simulink model "controller_modified_Ardiono"  (R2023b)
settings: Solver=FixedStepDiscrete  StartTime=0.0  StopTime=100  FixedStep=1/100  RelTol=1e-3  EnableMultiTasking=on
undefined symbols (not defined in the file): MAX_TORQUE, MAX_TORQUE_REVERSE
libraries: arduinolib x17
settings Model: ExtModeTrigDuration=2  Creator=DAUIN-Win10  LastModifiedBy=RSKALA
settings OptimizationCC: EnhancedBackFolding=on  PassReuseOutputArgsAs=Individual arguments  ZeroExternalMemoryAtStartup=off  ZeroInternalMemoryAtStartup=off  MaxStackSize=64  OptimizeBlockOrder=speed  DifferentSizesBufferReuse=on  OptimizationCustomize=off  EfficientTunableParamExpr=on
settings DebuggingCC: ParameterTunabilityLossMsg=error  UnconnectedInputMsg=warning  UnconnectedOutputMsg=warning  UnconnectedLineMsg=warning
settings HardwareCC: ProdBitPerInt=16  ProdBitPerPointer=16  ProdBitPerSizeT=16  ProdBitPerPtrDiffT=16  ProdLargestAtomicFloat=None  ProdWordSize=8  ProdHWDeviceType=Atmel->AVR
settings ModelReferenceCC: EnableRefExpFcnMdlSchedulingChecks=on
settings SFSimCC: MATLABDynamicMemAlloc=off
settings RTWCC: Description=Embedded Coder  SystemTargetFile=ert.tlc  HardwareBoard=Arduino Uno  TemplateMakefile=ert_default_tmf  Toolchain=Arduino AVR  BuildConfiguration=Faster Runs  DLArmComputeVersion=19.05
settings CodeAppCC: ForceParamTrailComments=on  IgnoreCustomStorageClasses=off  OperatorAnnotations=on  SimulinkDataObjDesc=on  SFDataObjDesc=on  InsertBlockDesc=on
settings ERTTargetCC: SupportContinuousTime=on  SupportVariableSizeSignals=on  ExtModeTransport=3  ExtModeStaticAlloc=on  ExtModeAutomaticAllocSize=off  ExtModeStaticAllocSize=250  ExtModeMexFile=ext_xcp  ExtModeIntrfLevel=Level2 - Open

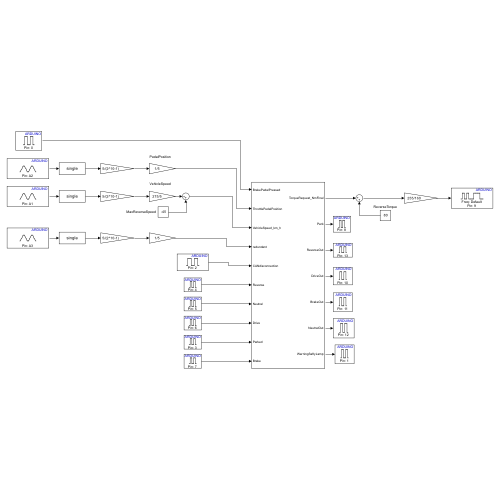
[thumbnail: Simulink's stored preview of the top-level diagram]
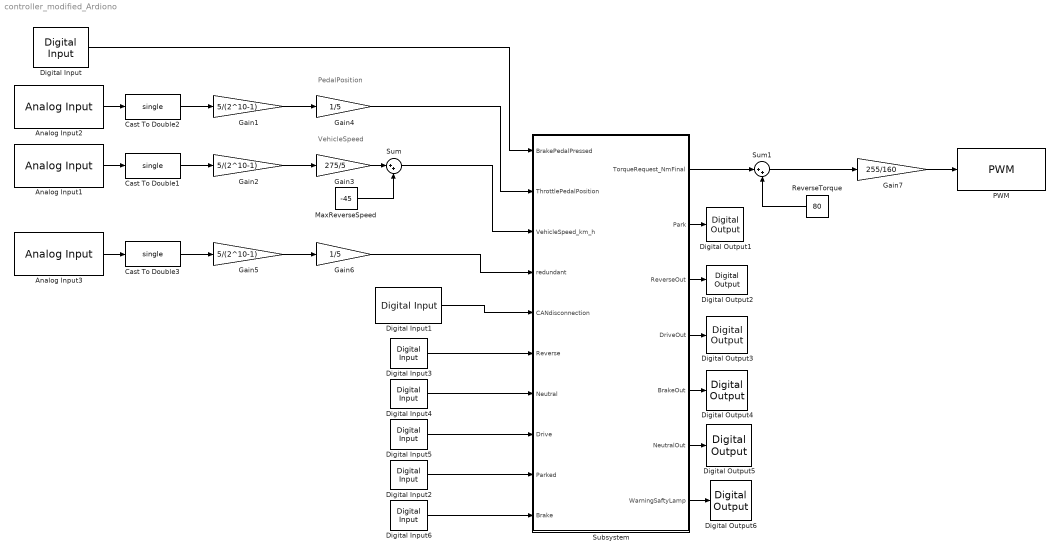
== system controller_modified_Ardiono ==
  note: VehicleSpeed
  note: PedalPosition
  Analog Input1 : arduinolib/Analog Input  pinNumber=1  ReadResultsOnly=off  ConversionTriggerSource=Software  ExternalTriggerType=uint32( 0 )  OutputDataType=uint16  EnableConversionCompleteNotify=off  EnableOuputStatus=off  SampleTime=-1  blockPlatform=arduino
  Analog Input2 : arduinolib/Analog Input  pinNumber=2  ReadResultsOnly=off  ConversionTriggerSource=Software  ExternalTriggerType=uint32( 0 )  OutputDataType=uint16  EnableConversionCompleteNotify=off  EnableOuputStatus=off  SampleTime=-1  blockPlatform=arduino
  Analog Input3 : arduinolib/Analog Input  pinNumber=3  ReadResultsOnly=off  ConversionTriggerSource=Software  ExternalTriggerType=uint32( 0 )  OutputDataType=uint16  EnableConversionCompleteNotify=off  EnableOuputStatus=off  SampleTime=-1  blockPlatform=arduino
  Cast To Double1 : DataTypeConversion  OutDataTypeStr=single  SaturateOnIntegerOverflow=off  RndMeth=Floor
  Cast To Double2 : DataTypeConversion  OutDataTypeStr=single  SaturateOnIntegerOverflow=off  RndMeth=Floor
  Cast To Double3 : DataTypeConversion  OutDataTypeStr=single  SaturateOnIntegerOverflow=off  RndMeth=Floor
  Digital Input : arduinolib/Digital Input  pinNumber=0  mode=Default  Direction=input  SampleTime=0.1  blockPlatform=arduino
  Digital Input1 : arduinolib/Digital Input  pinNumber=2  mode=Default  Direction=input  SampleTime=0.1  blockPlatform=arduino
  Digital Input2 : arduinolib/Digital Input  pinNumber=3  mode=Default  Direction=input  SampleTime=0.1  blockPlatform=arduino
  Digital Input3 : arduinolib/Digital Input  pinNumber=4  mode=Default  Direction=input  SampleTime=0.1  blockPlatform=arduino
  Digital Input4 : arduinolib/Digital Input  pinNumber=5  mode=Default  Direction=input  SampleTime=0.1  blockPlatform=arduino
  Digital Input5 : arduinolib/Digital Input  pinNumber=6  mode=Default  Direction=input  SampleTime=0.1  blockPlatform=arduino
  Digital Input6 : arduinolib/Digital Input  pinNumber=7  mode=Default  Direction=input  SampleTime=0.1  blockPlatform=arduino
  Digital Output1 : arduinolib/Digital Output  pinNumber=8  Direction=output  blockPlatform=arduino
  Digital Output2 : arduinolib/Digital Output  pinNumber=13  Direction=output  blockPlatform=arduino
  Digital Output3 : arduinolib/Digital Output  pinNumber=10  Direction=output  blockPlatform=arduino
  Digital Output4 : arduinolib/Digital Output  pinNumber=11  Direction=output  blockPlatform=arduino
  Digital Output5 : arduinolib/Digital Output  pinNumber=12  Direction=output  blockPlatform=arduino
  Digital Output6 : arduinolib/Digital Output  pinNumber=1  Direction=output  blockPlatform=arduino
  Gain1 : Gain  Gain=5/(2^10-1)
  Gain2 : Gain  Gain=5/(2^10-1)
  Gain3 : Gain  Gain=275/5  OutDataTypeStr=single
  Gain4 : Gain  Gain=1/5
  Gain5 : Gain  Gain=5/(2^10-1)
  Gain6 : Gain  Gain=1/5
  Gain7 : Gain  Gain=255/160
  MaxReverseSpeed : Constant  Value=-45  OutDataTypeStr=single
  PWM : arduinolib/PWM  pinNumber=9  frequencyType=Default  desiredFrequency=490.2  achievableFrequency=490.2
  ReverseTorque : Constant  Value=80
  Subsystem : Subsystem
  Sum : Sum  Inputs=|++  OutDataTypeStr=single
  Sum1 : Sum  Inputs=|++
  wires:
  Cast To Double2/1 -> Gain1/1
  Gain5/1 -> Gain6/1
  Digital Input3/1 -> Subsystem/6(Reverse)
  Analog Input2/1 -> Cast To Double2/1
  Gain2/1 -> Gain3/1
  Gain3/1 -> Sum/1
  MaxReverseSpeed/1 -> Sum/2
  Digital Input4/1 -> Subsystem/7(Neutral)
  Analog Input1/1 -> Cast To Double1/1
  Digital Input5/1 -> Subsystem/8(Drive)
  Analog Input3/1 -> Cast To Double3/1
  Digital Input6/1 -> Subsystem/10(Brake)
  Cast To Double3/1 -> Gain5/1
  Digital Input/1 -> Subsystem/1(BrakePedalPressed)
  Gain4/1 -> Subsystem/2(ThrottlePedalPosition)
  Sum/1 -> Subsystem/3(VehicleSpeed_km_h)
  Cast To Double1/1 -> Gain2/1
  Digital Input2/1 -> Subsystem/9(Parked)
  Gain1/1 -> Gain4/1
  Gain6/1 -> Subsystem/4(redundant)
  Digital Input1/1 -> Subsystem/5(CANdisconnection)
  Sum1/1 -> Gain7/1
  Gain7/1 -> PWM/1
  ReverseTorque/1 -> Sum1/2
  Subsystem/5(BrakeOut) -> Digital Output4/1
  Subsystem/4(DriveOut) -> Digital Output3/1
  Subsystem/3(ReverseOut) -> Digital Output2/1
  Subsystem/2(Park) -> Digital Output1/1
  Subsystem/1(TorqueRequest_NmFinal) -> Sum1/1
  Subsystem/6(NeutralOut) -> Digital Output5/1
  Subsystem/7(WarningSaftyLamp) -> Digital Output6/1

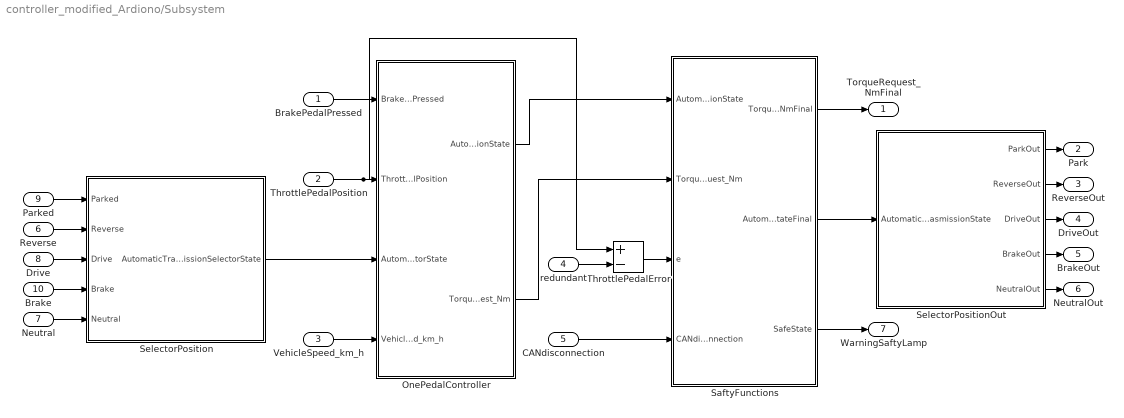
== system controller_modified_Ardiono/Subsystem ==
  BrakePedalPressed : Inport  OutDataTypeStr=boolean
  ThrottlePedalPosition : Inport  Port=2  OutDataTypeStr=single
  VehicleSpeed_km_h : Inport  Port=3  OutDataTypeStr=single  Unit=km/h
  redundant : Inport  Port=4  OutDataTypeStr=single  Unit=km/h
  CANdisconnection : Inport  Port=5
  Reverse : Inport  Port=6
  Neutral : Inport  Port=7
  Drive : Inport  Port=8
  Parked : Inport  Port=9
  Brake : Inport  Port=10
  OnePedalController : Stateflow chart  TreatAsAtomicUnit=on
  SaftyFunctions : Stateflow chart  TreatAsAtomicUnit=on
      settings: PortSchema="{\"entries\":[{\"content\":{\"sides\":[{\"content\":{\"connectorIds\":[\"In1\",\"In2\",\"In4\",\"In3\"]},\"type\":\"ConnectorPlacement.EquallySpacedRectSide\",\"uuid\":\"7fe74ee5-44b1-4d05-a413-f8cbf6cc4146\"},{\"content\":{\"connectorIds\":[\"Out1\",\"Out2\",\"Out3\"],\"side\":\"RIGHT\"},\"type\":\"ConnectorPlacement.EquallySpacedRectSide\",\"uuid\":\"213ffcbc-04cb-45d6-b82c-0aa6f7f2fafd\"},{\"content\":{\"side\":\"TOP\"},\"type\":\"ConnectorPlacement.EquallySpacedRectSide\",\"uuid\":\"fb1fe60a-13ea-4390-8839-03c13817aaf9\"},{\"content\":{\"side\":\"BOTTOM\"},\"type\":\"ConnectorPlacement.EquallySpacedRectSide\",\"uuid\":\"05eed5e2-92b4-4d65-939e-09ec5391c094\"}]},\"type\":\"ConnectorPlacement.EquallySpacedConnector\",\"uuid\":\"3e98ccd8-4ab9-4b74-b636-0629ec9fe3f2\"}],\"packageUris\":[\"http://schema.mathworks.com/mf0/Connector/R2020b\"],\"version\":\"1.0\"}"
  SelectorPosition : Stateflow chart  TreatAsAtomicUnit=on
  SelectorPositionOut : Stateflow chart  TreatAsAtomicUnit=on
  ThrottlePedalError : Sum  Inputs=+-
  TorqueRequest_NmFinal : Outport  OutDataTypeStr=single  Unit=N*m
  Park : Outport  Port=2  OutDataTypeStr=single  Unit=N*m
  ReverseOut : Outport  Port=3  OutDataTypeStr=single  Unit=N*m
  DriveOut : Outport  Port=4  OutDataTypeStr=single  Unit=N*m
  BrakeOut : Outport  Port=5  OutDataTypeStr=single  Unit=N*m
  NeutralOut : Outport  Port=6  OutDataTypeStr=single  Unit=N*m
  WarningSaftyLamp : Outport  Port=7
  wires:
  ThrottlePedalPosition/1 -> OnePedalController/2(ThrottlePedalPosition), ThrottlePedalError/1
  SaftyFunctions/1(TorqueRequest_NmFinal) -> TorqueRequest_NmFinal/1
  BrakePedalPressed/1 -> OnePedalController/1(BrakePedalPressed)
  SelectorPosition/1(AutomaticTrasmissionSelectorState) -> OnePedalController/3(AutomaticTrasmissionSelectorState)
  VehicleSpeed_km_h/1 -> OnePedalController/4(VehicleSpeed_km_h)
  CANdisconnection/1 -> SaftyFunctions/3(CANdisconnection)
  SaftyFunctions/2(AutomaticTransmissionStateFinal) -> SelectorPositionOut/1(AutomaticTrasmissionState)
  redundant/1 -> ThrottlePedalError/2
  ThrottlePedalError/1 -> SaftyFunctions/4(e)
  OnePedalController/1(AutomaticTransmissionState) -> SaftyFunctions/1(AutomaticTransmissionState)
  OnePedalController/2(TorqueRequest_Nm) -> SaftyFunctions/2(TorqueRequest_Nm)
  SaftyFunctions/3(SafeState) -> WarningSaftyLamp/1
  SelectorPositionOut/3(DriveOut) -> DriveOut/1
  SelectorPositionOut/1(ParkOut) -> Park/1
  SelectorPositionOut/4(BrakeOut) -> BrakeOut/1
  SelectorPositionOut/2(ReverseOut) -> ReverseOut/1
  SelectorPositionOut/5(NeutralOut) -> NeutralOut/1
  Drive/1 -> SelectorPosition/3(Drive)
  Reverse/1 -> SelectorPosition/2(Reverse)
  Parked/1 -> SelectorPosition/1(Parked)
  Neutral/1 -> SelectorPosition/5(Neutral)
  Brake/1 -> SelectorPosition/4(Brake)

== stateflow chart controller_modified_Ardiono/Subsystem/SelectorPositionOut ==
  state init1
  state P
    en:
    ParkOut=1
    ex:
    ParkOut=0
  state B
    en:
    BrakeOut=1
    ex:
    BrakeOut=0
  state R
    en:
    ReverseOut=1
    ex:
    ReverseOut=0
  state N
    en:
    NeutralOut=1
    ex:
    NeutralOut=0
  state D
    en:
    DriveOut=1
    ex:
    DriveOut=0
  (default) -> init1
  P -> init1 : [AutomaticTrasmissionState~=TransmissionState.Park]
  init1 -> P [order 5] : [AutomaticTrasmissionState==TransmissionState.Park]
  init1 -> B [order 1] : [AutomaticTrasmissionState==TransmissionState.Brake]
  B -> init1 : [AutomaticTrasmissionState~=TransmissionState.Brake]
  R -> init1 : [AutomaticTrasmissionState~=TransmissionState.Reverse]
  init1 -> R [order 4] : [AutomaticTrasmissionState==TransmissionState.Reverse]
  N -> init1 : [AutomaticTrasmissionState~=TransmissionState.Neutral]
  init1 -> N [order 3] : [AutomaticTrasmissionState==TransmissionState.Neutral]
  init1 -> D [order 2] : [AutomaticTrasmissionState==TransmissionState.Drive]
  D -> init1 : [AutomaticTrasmissionState~=TransmissionState.Drive]
  data: AutomaticTrasmissionState input Enum: TransmissionState; ParkOut output single; ReverseOut output single; DriveOut output single; BrakeOut output single; NeutralOut output single

== stateflow chart controller_modified_Ardiono/Subsystem/SaftyFunctions ==
  state StateStateON
    du:
    AutomaticTransmissionStateFinal=TransmissionState.Neutral
    TorqueRequest_NmFinal=0
    SafeState=1
  state init
  state SafeStateOFF
    du:
    TorqueRequest_NmFinal=TorqueRequest_Nm
    AutomaticTransmissionStateFinal=AutomaticTransmissionState
    SafeState=0
  (default) -> init
  init -> StateStateON [order 2] : [e~=0 ||CANdisconnection==1 ]
  StateStateON -> init : [e==0&&CANdisconnection==0]
  init -> SafeStateOFF [order 1] : [e==0&&CANdisconnection==0]
  SafeStateOFF -> init : [e~=0||CANdisconnection==1]
  data: AutomaticTransmissionState input; TorqueRequest_Nm input; CANdisconnection input; e input; TorqueRequest_NmFinal output; AutomaticTransmissionStateFinal output; SafeState output

== stateflow chart controller_modified_Ardiono/Subsystem/OnePedalController ==
  state P
    en:
    AutomaticTransmissionState=TransmissionState.Park;
    du:
    TorqueRequest_Nm=0;
  state B
    en:
    AutomaticTransmissionState=TransmissionState.Brake;
    state Accelerate
      du:
      TorqueRequest_Nm=MAX_TORQUE*(3/2)*(ThrottlePedalPosition-(1/3));
    state Stop
      en:
      TorqueRequest_Nm=0;
    state Decelerate
      du:
      TorqueRequest_Nm=-MAX_TORQUE*(1-3*ThrottlePedalPosition);
    (default) -> Accelerate
    Stop -> Accelerate : [ThrottlePedalPosition>=1/3]
    Accelerate -> Decelerate : [ThrottlePedalPosition<=(1/3)]
    Decelerate -> Accelerate [order 2] : [ThrottlePedalPosition>(1/3)]
    Decelerate -> Stop [order 1] : [VehicleSpeed_km_h<=0]
  state N
    en:
    AutomaticTransmissionState=TransmissionState.Neutral;
    du:
    TorqueRequest_Nm=0;
  state R
    en:
    AutomaticTransmissionState=TransmissionState.Reverse;
    du:
    TorqueRequest_Nm=ThrottlePedalPosition*-MAX_TORQUE_REVERSE;
  state D
    en:
    AutomaticTransmissionState=TransmissionState.Drive;
    du:
    TorqueRequest_Nm=ThrottlePedalPosition*MAX_TORQUE;
  (default) -> P
  P -> N : [AutomaticTrasmissionSelectorState~=TransmissionState.Park&BrakePedalPressed==1]
  N -> P [order 1] : [AutomaticTrasmissionSelectorState==TransmissionState.Park&BrakePedalPressed==1&abs(VehicleSpeed_km_h)<5]
  N -> D [order 2] : [( AutomaticTrasmissionSelectorState==TransmissionState.Drive||AutomaticTrasmissionSelectorState==TransmissionState.Brake)&BrakePedalPressed==1&VehicleSpeed_km_h>-5]
  R -> N : [AutomaticTrasmissionSelectorState~=TransmissionState.Reverse]
  D -> N [order 2] : [AutomaticTrasmissionSelectorState==TransmissionState.Neutral || AutomaticTrasmissionSelectorState==TransmissionState.Reverse || AutomaticTrasmissionSelectorState==TransmissionState.Park]
  D -> B [order 1] : [ ThrottlePedalPosition>(1/3)&AutomaticTrasmissionSelectorState==TransmissionState.Brake]
  N -> R [order 3] : [AutomaticTrasmissionSelectorState==TransmissionState.Reverse&BrakePedalPressed==1&VehicleSpeed_km_h<5]
  B -> D : [AutomaticTrasmissionSelectorState~=TransmissionState.Brake]
  data: BrakePedalPressed input boolean; ThrottlePedalPosition input single; AutomaticTrasmissionSelectorState input Enum: TransmissionState; VehicleSpeed_km_h input single; AutomaticTransmissionState output Enum: TransmissionState; TorqueRequest_Nm output single; MAX_TORQUE_REVERSE parameter; MAX_TORQUE parameter

== stateflow chart controller_modified_Ardiono/Subsystem/SelectorPosition ==
  state init
  state P
    en:
    AutomaticTrasmissionSelectorState=TransmissionState.Park
  state B
    en:
    AutomaticTrasmissionSelectorState=TransmissionState.Brake
  state R
    en:
    AutomaticTrasmissionSelectorState=TransmissionState.Reverse
  state N
    en:
    AutomaticTrasmissionSelectorState=TransmissionState.Neutral
  state D
    en:
    AutomaticTrasmissionSelectorState=TransmissionState.Drive
  (default) -> init
  P -> init : [Parked~=1]
  init -> P [order 5] : [Parked==1]
  init -> B [order 1] : [Brake==1]
  B -> init : [Brake~=1]
  R -> init : [Reverse~=1]
  init -> R [order 4] : [Reverse==1]
  N -> init : [Neutral~=1]
  init -> N [order 3] : [Neutral==1]
  init -> D [order 2] : [Drive==1]
  D -> init : [Drive~=1]
  data: AutomaticTrasmissionSelectorState output Enum: TransmissionState; Parked input; Reverse input; Drive input; Brake input; Neutral input
